simulink model "FlexLink_ExciteMode"  (Simulink 10.0)
settings: Solver=ode1  StartTime=0.0  StopTime=60  FixedStep=0.002  RelTol=1e-3  EnableMultiTasking=on
undefined symbols (not defined in the file): HIL, qc_get_step_size
libraries: quarc_library x5, simulink_extras x2, simulink x1
settings Model: Creator=MLevis  LastModifiedBy=dgweon6  SimulationMode=external  ExtModeTrigDuration=30001
settings SolverCC: PositivePriorityOrder=on
settings DataIOCC: SignalLoggingSaveFormat=ModelDataLogs
settings OptimizationCC: BooleanDataType=off  OptimizeBlockIOStorage=off  BufferReuse=off  GlobalBufferReuse=off  ExpressionFolding=off  ExpressionDepthLimit=2147483647  LocalBlockOutputs=off  InitFltsAndDblsToZero=on  OptimizeDataStoreBuffers=off  BusAssignmentInplaceUpdate=off
settings DebuggingCC: SaveWithParameterizedLinksMsg=none  SignalResolutionControl=TryResolveAllWithWarning  MultiTaskDSMMsg=warning  MultiTaskCondExecSysMsg=none  FcnCallInpInsideContextMsg=warning  StateNameClashWarn=warning
settings RTWCC: Description=QUARC Win64 Target  SystemTargetFile=quarc_win64.tlc  TemplateMakefile=quarc_default_tmf
settings STFCustomTargetCC: TargetPreCompLibLocation=C:\PROGRA~3\QUARC\lib\2019b\win64\release  ConcurrentExecutionCompliant=on  GeneratePreprocessorConditionals=Disable all  CombineOutputUpdateFcns=on  CPPClassGenCompliant=on  GRTInterface=off  SystemTargetFile=quarc_win64.tlc
settings GRTTargetCC: TargetPreCompLibLocation=C:\PROGRA~3\QUARC\lib\2019b\win64\release  ParMdlRefBuildCompliant=off  CompOptLevelCompliant=off  GeneratePreprocessorConditionals=Disable all  CombineOutputUpdateFcns=on  MatFileLogging=off  GRTInterface=off  UseToolchainInfoCompliant=off  ExtMode=on  ExtModeMexFile=quarc_comm
settings ConfigComp: CovExternalEMLEnable=off

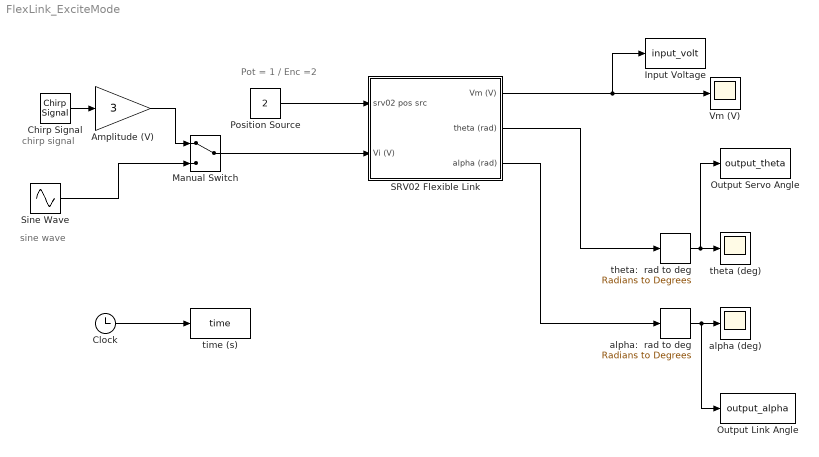
== system FlexLink_ExciteMode ==
  note: sine wave
  note: chirp signal
  note: Pot = 1 / Enc =2
  Amplitude (V) : Gain  Gain=3  SaturateOnIntegerOverflow=on  OutDataTypeStr=Inherit: Same as input  ParamDataTypeStr=Inherit: Same as input
  Chirp Signal : simulink/Sources/Chirp Signal  f1=0.1  T=0.25  f2=0.2
  Clock : Clock
  Input Voltage : ToWorkspace  VariableName=input_volt  SampleTime=-1
  Manual Switch : ManualSwitch
  Output Link Angle : ToWorkspace  VariableName=output_alpha  SampleTime=-1
  Output Servo Angle : ToWorkspace  VariableName=output_theta  SampleTime=-1
  Position Source : Constant  Value=2
  SRV02 Flexible Link : Subsystem
  Sine Wave : Sin  Amplitude=3  Frequency=0  SampleTime=0
  Vm (V) : Scope
  alpha (deg) : Scope
  alpha:  rad to deg : simulink_extras/Transformations/Radians to Degrees
  theta (deg) : Scope
  theta:  rad to deg : simulink_extras/Transformations/Radians to Degrees
  time (s) : ToWorkspace  VariableName=time  SampleTime=-1
  wires:
  Position Source/1 -> SRV02 Flexible Link/1(srv02 pos src)
  theta:  rad to deg/1 -> Output Servo Angle/1, theta (deg)/1
  alpha:  rad to deg/1 -> Output Link Angle/1, alpha (deg)/1
  Manual Switch/1 -> SRV02 Flexible Link/2(Vi (V))
  Amplitude (V)/1 -> Manual Switch/1
  Sine Wave/1 -> Manual Switch/2
  SRV02 Flexible Link/1(Vm (V)) -> Input Voltage/1, Vm (V)/1
  SRV02 Flexible Link/3(alpha (rad)) -> alpha:  rad to deg/1
  Chirp Signal/1 -> Amplitude (V)/1
  SRV02 Flexible Link/2(theta (rad)) -> theta:  rad to deg/1
  Clock/1 -> time (s)/1

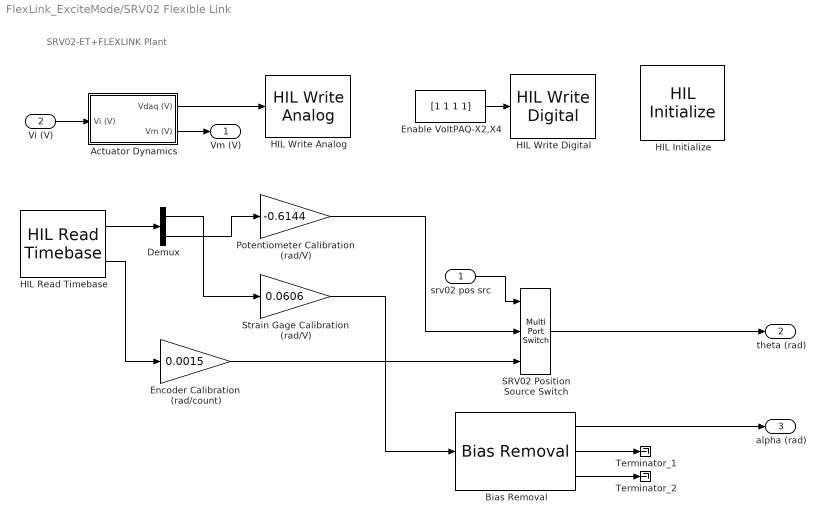
== system FlexLink_ExciteMode/SRV02 Flexible Link ==
  note: SRV02-ET+FLEXLINK Plant
  srv02 pos src : Inport
  Vi (V) : Inport  Port=2
  Actuator Dynamics : Subsystem
  Bias Removal : quarc_library/Discrete/Bias Removal  start_time=0  end_time=0.1  switch_id=0  sample_time=qc_get_step_size
      settings: SourceProductName=QUARC Targets
  Demux : Demux  Outputs=2
  Enable VoltPAQ-X2,X4 : Constant  Value=[1 1 1 1]
  Encoder Calibration  (rad/count) : Gain  Gain=0.0015  SaturateOnIntegerOverflow=on  OutDataTypeStr=Inherit: Same as input  ParamDataTypeStr=Inherit: Same as input
  HIL Initialize : quarc_library/Data Acquisition/Generic/Configuration/HIL Initialize  object_name=HIL-1  board_type=q2_usb  board_number=0  board_options=d0=digital;d1=digital;led=auto;update_rate=normal;decimation=1  exclusive=off  active=off  hardware_clocks=[0:2]  clock_modes=[]  initial_clock_frequencies=[]  set_clock_params_at_start=off  set_clock_params_at_switch_in=off  set_clock_frequencies_at_start=off  set_clock_frequencies_at_switch_in=off  analog_input_channels=[0:1]  analog_input_configurations=[]  analog_input_maximums=10  analog_input_minimums=-10  set_analog_input_params_at_start=on  set_analog_input_params_at_switch_in=off  analog_output_channels=[0:1]  analog_output_maximums=10  analog_output_minimums=-10  initial_analog_outputs=[0]  final_analog_outputs=[0]  watchdog_analog_outputs=0  set_analog_output_params_at_start=on  set_analog_output_params_at_switch_in=off  set_analog_outputs_at_start=on  set_analog_outputs_at_switch_in=off  set_analog_outputs_at_terminate=on  set_analog_outputs_at_switch_out=off  set_analog_outputs_on_watchdog=off  digital_input_channels=[]  digital_output_channels=[]  digital_output_configuration=[]  initial_digital_outputs=[1]  final_digital_outputs=[1]  watchdog_digital_outputs=[1]  set_digital_output_params_at_start=off  set_digital_output_params_at_switch_in=off  set_digital_outputs_at_start=on  set_digital_outputs_at_switch_in=off  set_digital_outputs_at_terminate=on  set_digital_outputs_at_switch_out=off  set_digital_outputs_on_watchdog=off  encoder_channels=[0:1]  quadrature=[4]  encoder_filter_frequency=[]  initial_encoder_counts=[0]  set_encoder_params_at_start=on  set_encoder_params_at_switch_in=off  set_encoder_counts_at_start=on  set_encoder_counts_at_switch_in=off  pwm_channels=[]  pwm_modes=0  pwm_frequency=1/0.020  pwm_configuration=[0]  pwm_alignment=[0]  pwm_polarity=[1]  pwm_leading_deadband=[0]  pwm_trailing_deadband=[0]  initial_pwm_outputs=[0]  final_pwm_outputs=[0]  watchdog_pwm_outputs=[0]  set_pwm_params_at_start=on  set_pwm_params_at_switch_in=off  set_pwm_outputs_at_start=on  set_pwm_outputs_at_switch_in=off  set_pwm_outputs_at_terminate=on  set_pwm_outputs_at_switch_out=off  set_pwm_outputs_on_watchdog=off  other_output_channels=[]  initial_other_outputs=[]  final_other_outputs=[]  watchdog_other_outputs=[]  set_other_outputs_at_start=off  set_other_outputs_at_switch_in=off  set_other_outputs_at_terminate=off  set_other_outputs_at_switch_out=off  set_other_outputs_on_watchdog=off
  HIL Read Timebase : quarc_library/Data Acquisition/Generic/Timebases/HIL Read Timebase  object_name=HIL-1  clock=0  analog_channels=[0:1]  encoder_channels=[0]  digital_channels=[]  other_channels=[]  samples_in_buffer=max(ceil(1/qc_get_step_size), 1)  active=on  vector_output=on  data_type_mode=Inherit via back propagation  encoder_data_type=double  digital_data_type=boolean
  HIL Write Analog : quarc_library/Data Acquisition/Generic/Immediate I//O/HIL Write Analog  object_name=HIL-1  channels=0  sample_time=-1  active=off  vector_input=off
  HIL Write Digital : quarc_library/Data Acquisition/Generic/Immediate I//O/HIL Write Digital  object_name=HIL-1  channels=[0:3]  sample_time=-1  active=off  vector_input=on
      settings: SourceProductName=QUARC Targets
  Potentiometer Calibration  (rad/V) : Gain  Gain=-0.6144  SaturateOnIntegerOverflow=on  OutDataTypeStr=Inherit: Same as input  ParamDataTypeStr=Inherit: Same as input
  SRV02 Position Source Switch : MultiPortSwitch  Inputs=2
  Strain Gage Calibration  (rad/V) : Gain  Gain=0.0606  SaturateOnIntegerOverflow=on  OutDataTypeStr=Inherit: Same as input  ParamDataTypeStr=Inherit: Same as input
  Terminator_1 : Terminator
  Terminator_2 : Terminator
  Vm (V) : Outport  InitialOutput=0  VectorParamsAs1DForOutWhenUnconnected=off
  theta (rad) : Outport  Port=2  InitialOutput=0  VectorParamsAs1DForOutWhenUnconnected=off
  alpha (rad) : Outport  Port=3  InitialOutput=0  VectorParamsAs1DForOutWhenUnconnected=off
  wires:
  Potentiometer Calibration  (rad/V)/1 -> SRV02 Position Source Switch/2
  HIL Read Timebase/1 -> Demux/1
  Encoder Calibration  (rad/count)/1 -> SRV02 Position Source Switch/3
  HIL Read Timebase/2 -> Encoder Calibration  (rad/count)/1
  srv02 pos src/1 -> SRV02 Position Source Switch/1
  Actuator Dynamics/2(Vm (V)) -> Vm (V)/1
  Actuator Dynamics/1(Vdaq (V)) -> HIL Write Analog/1
  Vi (V)/1 -> Actuator Dynamics/1(Vi (V))
  Enable VoltPAQ-X2,X4/1 -> HIL Write Digital/1
  Bias Removal/2 -> Terminator_1/1
  Bias Removal/3 -> Terminator_2/1
  SRV02 Position Source Switch/1 -> theta (rad)/1
  Demux/1 -> Strain Gage Calibration  (rad/V)/1
  Demux/2 -> Potentiometer Calibration  (rad/V)/1
  Strain Gage Calibration  (rad/V)/1 -> Bias Removal/1
  Bias Removal/1 -> alpha (rad)/1

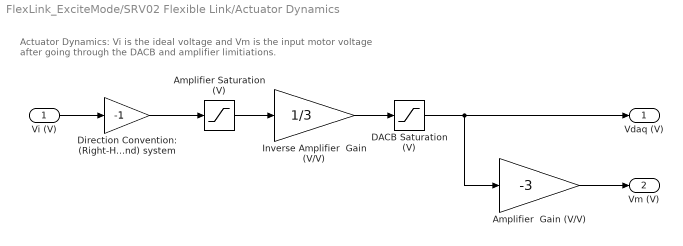
== system FlexLink_ExciteMode/SRV02 Flexible Link/Actuator Dynamics ==
  note: Actuator Dynamics: Vi is the ideal voltage and Vm is the
      | input motor voltage after going through the DACB and amplifier limitiations.
  Vi (V) : Inport
  Amplifier Saturation (V) : Saturate  UpperLimit=24  LowerLimit=-24
  Amplifier  Gain (V/V) : Gain  Gain=-3
  DACB Saturation (V) : Saturate  UpperLimit=10  LowerLimit=-10
  Direction Convention: (Right-Hand) system : Gain  Gain=-1  SaturateOnIntegerOverflow=on  OutDataTypeStr=Inherit: Same as input  ParamDataTypeStr=Inherit: Same as input
  Inverse Amplifier  Gain (V/V) : Gain  Gain=1/3
  Vdaq (V) : Outport  VectorParamsAs1DForOutWhenUnconnected=off
  Vm (V) : Outport  Port=2  VectorParamsAs1DForOutWhenUnconnected=off
  wires:
  Direction Convention: (Right-Hand) system/1 -> Amplifier Saturation (V)/1
  Amplifier  Gain (V/V)/1 -> Vm (V)/1
  DACB Saturation (V)/1 -> Vdaq (V)/1, Amplifier  Gain (V/V)/1
  Inverse Amplifier  Gain (V/V)/1 -> DACB Saturation (V)/1
  Amplifier Saturation (V)/1 -> Inverse Amplifier  Gain (V/V)/1
  Vi (V)/1 -> Direction Convention: (Right-Hand) system/1
